simulink model "GHV_open_air_ang_trajectory_design_equation"  (R2023b)
settings: Solver=VariableStepAuto  StartTime=0.0  StopTime=130  FixedStep=0.0000001  MaxStep=0.1
undefined symbols (not defined in the file or in its folder): GHV_cfg, Ma, vc
libraries: simulink_extras x2
settings Model: SimulationMode=accelerator  Creator=Admin  LastModifiedBy=Admin

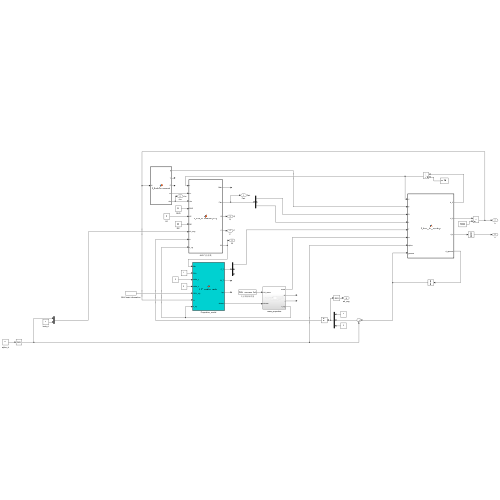
[thumbnail: Simulink's stored preview of the top-level diagram]
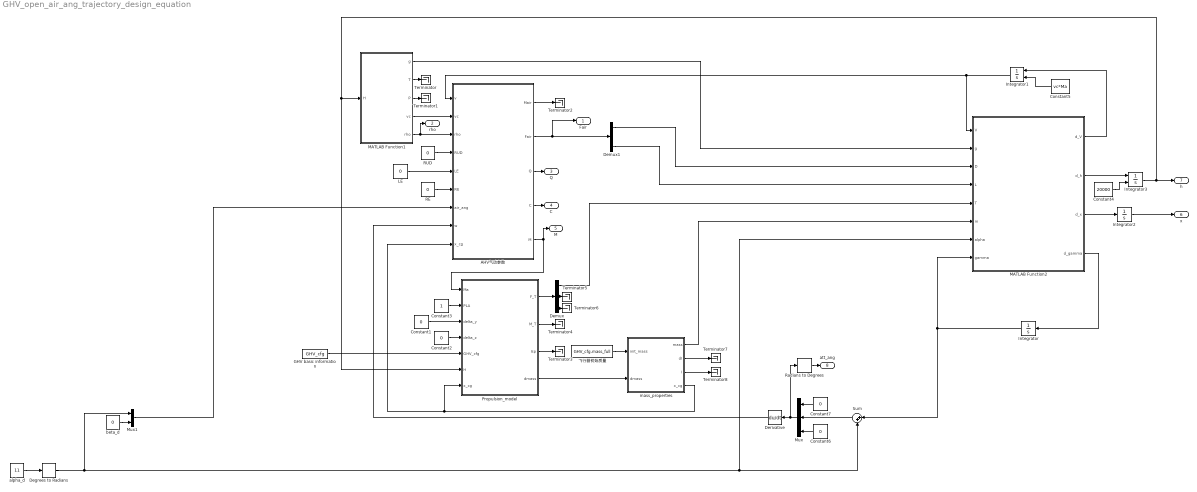
== system GHV_open_air_ang_trajectory_design_equation ==
  AHV气动参数 : MATLAB Function  TreatAsAtomicUnit=on
  Constant{1..2,6..7} (4 alike) : Constant  Value=0
  Constant3 : Constant
  Constant4 : Constant  Value=20000
  Constant5 : Constant  Value=vc*Ma
  Degrees to Radians : simulink_extras/Transformations/Degrees to Radians
  Demux : Demux  Outputs=3
  Demux1 : Demux  Outputs=3
  Derivative : Derivative
  GHV basic information : Constant  Value=GHV_cfg  VectorParams1D=off  OutDataTypeStr=Bus: slBus1
  Integrator : Integrator
  Integrator1 : Integrator  InitialConditionSource=external
  Integrator2 : Integrator
  Integrator3 : Integrator  InitialConditionSource=external
  LE : Constant  Value=0
  MATLAB Function1 : MATLAB Function  TreatAsAtomicUnit=on
  MATLAB Function2 : MATLAB Function  TreatAsAtomicUnit=on
  Mux : Mux  Inputs=3
  Mux1 : Mux  Inputs=2
  Propulsion_model : MATLAB Function  TreatAsAtomicUnit=on
  RE : Constant  Value=0
  RUD : Constant  Value=0
  Radians to Degrees : simulink_extras/Transformations/Radians to Degrees
  Sum : Sum  Inputs=|++
  Terminator{,1..8} (9 alike) : Terminator
  alpha_d : Constant  Value=11
  beta_d : Constant  Value=0
  mass_properties : Subsystem
  飞行器初始质量 : Constant  Value=GHV_cfg.mass_full
  Fair : Outport  SignalName=Fair
  rho : Outport  Port=2  SignalName=rho
  Q : Outport  Port=3  SignalName=Q
  C : Outport  Port=4  SignalName=C
  M : Outport  Port=5
  x : Outport  Port=6
  h : Outport  Port=7
  att_ang : Outport  Port=8
  wires:
  AHV气动参数/2(Fair) -> Demux1/1, Fair/1
  MATLAB Function1/5(rho) -> rho/1, AHV气动参数/3(rho)
  MATLAB Function1/4(vc) -> AHV气动参数/2(vc)
  MATLAB Function1/1(g) -> MATLAB Function2/2(g)
  RUD/1 -> AHV气动参数/4(RUD)
  AHV气动参数/5(M) -> Propulsion_model/1(Ma), M/1
  AHV气动参数/3(Q) -> Q/1
  AHV气动参数/4(C) -> C/1
  RE/1 -> AHV气动参数/6(RE)
  LE/1 -> AHV气动参数/5(LE)
  MATLAB Function1/2(T) -> Terminator/1
  MATLAB Function1/3(P) -> Terminator1/1
  飞行器初始质量/1 -> mass_properties/1(init_mass)
  Propulsion_model/4(dmass) -> mass_properties/2(dmass)
  Propulsion_model/3(Isp) -> Terminator3/1
  Propulsion_model/2(M_T) -> Terminator4/1
  mass_properties/1(mass) -> MATLAB Function2/6(m)
  Propulsion_model/1(F_T) -> Demux/1
  Demux/2 -> Terminator5/1
  Demux/3 -> Terminator6/1
  Demux/1 -> MATLAB Function2/5(T)
  mass_properties/4(x_cg) -> AHV气动参数/9(x_cg), Propulsion_model/7(x_cg)
  mass_properties/2(dI) -> Terminator7/1
  mass_properties/3(I) -> Terminator8/1
  GHV basic information/1 -> Propulsion_model/5(GHV_cfg)
  Constant2/1 -> Propulsion_model/4(delta_z)
  Constant1/1 -> Propulsion_model/3(delta_y)
  AHV气动参数/1(Mair) -> Terminator2/1
  Constant3/1 -> Propulsion_model/2(PLA)
  Demux1/1 -> MATLAB Function2/3(D)
  Demux1/3 -> MATLAB Function2/4(L)
  MATLAB Function2/4(d_gamma) -> Integrator/1
  Integrator/1 -> Sum/1, MATLAB Function2/8(gamma)
  MATLAB Function2/1(d_V) -> Integrator1/1
  Integrator1/1 -> MATLAB Function2/1(V), AHV气动参数/1(v)
  MATLAB Function2/2(d_h) -> Integrator3/1
  MATLAB Function2/3(d_x) -> Integrator2/1
  Integrator2/1 -> x/1
  Integrator3/1 -> Propulsion_model/6(H), MATLAB Function1/1(H), h/1
  Constant4/1 -> Integrator3/2
  Constant5/1 -> Integrator1/2
  Constant6/1 -> Mux/3
  Constant7/1 -> Mux/1
  alpha_d/1 -> Degrees to Radians/1
  Sum/1 -> Mux/2
  Degrees to Radians/1 -> Mux1/1, Sum/2, MATLAB Function2/7(alpha)
  beta_d/1 -> Mux1/2
  Mux1/1 -> AHV气动参数/7(air_ang)
  Mux/1 -> Radians to Degrees/1, Derivative/1
  Derivative/1 -> AHV气动参数/8(w)
  Radians to Degrees/1 -> att_ang/1

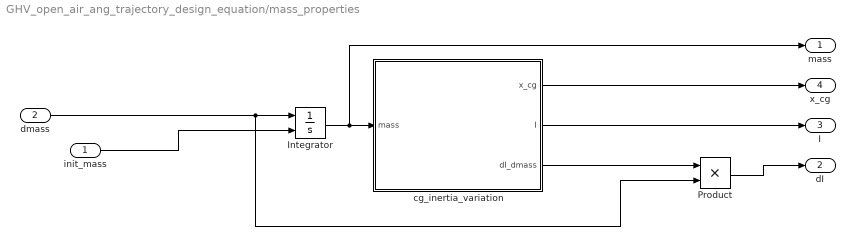
== system GHV_open_air_ang_trajectory_design_equation/mass_properties ==
  init_mass : Inport
  dmass : Inport  Port=2
  Integrator : Integrator  InitialConditionSource=external
  Product : Product
  cg_inertia_variation : MATLAB Function  TreatAsAtomicUnit=on
  mass : Outport
  dI : Outport  Port=2
  I : Outport  Port=3
  x_cg : Outport  Port=4
  wires:
  Integrator/1 -> mass/1, cg_inertia_variation/1(mass)
  init_mass/1 -> Integrator/2
  cg_inertia_variation/3(dI_dmass) -> Product/1
  dmass/1 -> Product/2, Integrator/1
  cg_inertia_variation/2(I) -> I/1
  cg_inertia_variation/1(x_cg) -> x_cg/1
  Product/1 -> dI/1

== matlab function GHV_open_air_ang_trajectory_design_equation/MATLAB Function2 ==
  data: V input; d_V output; d_h output; g input; D input; L input; d_x output; d_gamma output; T input; m input; alpha input; gamma input
function [d_V, d_h, d_x, d_gamma] = S_three_dof_trajectory(V, g, D, L, T, m, alpha, gamma)

    [d_V, d_gamma, d_x, d_h] = three_dof_trajectory(T, D, L, alpha, m, g, V, gamma);


end

== matlab function GHV_open_air_ang_trajectory_design_equation/AHV气动参数 ==
  data: Mair output; Fair output; Q output; C output; M output; v input; vc input; rho input; RUD input; LE input; RE input; air_ang input; w input; x_cg input
function [Mair, Fair, Q, C, M] = S_Get_Aerodynamic_xcg(v, vc, rho, RUD, LE, RE, air_ang, w, x_cg)

    Fair = zeros(3, 1);
    Mair = zeros(3, 1);
    C = zeros(6, 1);
    M = zeros(1, 1);
    Q = zeros(1, 1);

[M, Fair, Mair, Q, C] = Get_Aerodynamic_xcg(LE, RE, RUD, air_ang, v, w, vc, rho, x_cg);
   
end

== matlab function GHV_open_air_ang_trajectory_design_equation/MATLAB Function1 ==
  data: g output; H input; T output; P output; vc output; rho output
function [g, T, P, vc, rho] = S_EarthEnvironment(H)

[T, vc, P, rho, g] = EarthEnvironment(H);

end

== matlab function GHV_open_air_ang_trajectory_design_equation/Propulsion_model ==
  data: Ma input; PLA input; delta_y input; delta_z input; GHV_cfg input; H input; F_T output; M_T output; x_cg input; Isp output; dmass output
function [F_T,M_T, Isp,  dmass] = S_Propulsion_model(Ma, PLA, delta_y, delta_z, GHV_cfg, H, x_cg)
    F_T = zeros(3, 1); %#ok<PREALL>
    M_T = zeros(3, 1); %#ok<PREALL>
   [F_T, M_T, Isp, dmass] = Propulsion_model(PLA, H, Ma, delta_y, delta_z, GHV_cfg, x_cg);

end

== matlab function GHV_open_air_ang_trajectory_design_equation/mass_properties/cg_inertia_variation ==
  data: mass input; x_cg output; I output; dI_dmass output
function [x_cg, I, dI_dmass] = S_cg_inertia_variation(mass)

     [x_cg, I, dI_dmass] = cg_inertia_variation(mass);
     
end
